simulink model "SS_Flyback_PLECS_Model_EVAL2"  (R2019b)
settings: Solver=VariableStepAuto  StartTime=0.0  StopTime=Ts  RelTol=1e-3
undefined symbols (not defined in the file or in its folder): fixed, plecs
libraries: plecslib_extras2 x1
settings Model: Creator=jbaxte24  LastModifiedBy=jb
settings DataIOCC: ReturnWorkspaceOutputs=off
settings DebuggingCC: ArithmeticOperatorsInVariantConditions=warning
settings SFSimCC: SimUseLocalCustomCode=off  CustomCodeUndefinedFunction=UseInterfaceOnly
settings RTWCC: RTWUseLocalCustomCode=off
settings CodeAppCC: StateflowObjectComments=on

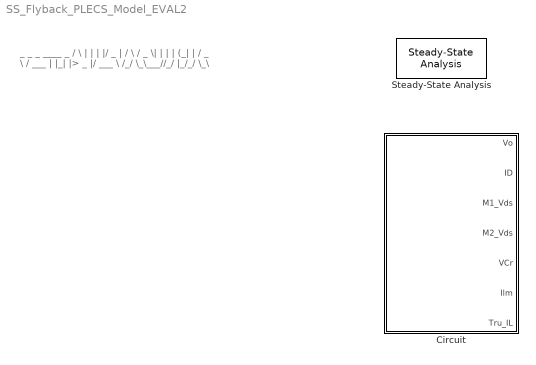
== system SS_Flyback_PLECS_Model_EVAL2 ==
  note: _ _ _ ____ _
      | / \ | | | |/ _ | / \
      | / _ \| | | | (_| | / _ \
      | / ___ | |_| |> _ |/ ___ \
      | /_/ \_\___//_/ |_/_/ \_\
  Circuit : Subsystem  LoadFcn=plecs('sl', 200);  InitFcn=plecs('sl', 214);  StartFcn=plecs('sl', 208);  StopFcn=plecs('sl', 209);  mask(PlecsCircuit){PLECSData=<binary blob, 3564 chars, not shown>}
      mask prompts: PLECSData "PLECS Data (Do not delete or modify!)"
      mask init:
      | % PLACE CUSTOM INITIALIZATIONS ABOVE
      | % DO NOT REMOVE
      | plecs('sl', 215);
      | % DO NOT REMOVE
      settings: CopyFcn=plecs('sl', 203);  DeleteFcn=plecs('sl', 205);  UndoDeleteFcn=plecs('sl', 206);  PreSaveFcn=plecs('sl', 211);  PostSaveFcn=plecs('sl', 201);  NameChangeFcn=plecs('sl', 210);  DestroyFcn=plecs('sl', 207);  PreCopyFcn=plecs('sl', 216);  OpenFcn=plecs('sl', 202);  ErrorFcn=plerrorfcn
      mask Help: web(['file:///' fullfile(plecsdoc, 'creatingacircuit.html')])
      mask Display: disp('PLECS\nCircuit')
  Steady-State Analysis : plecslib_extras2/Analysis Tools/Steady-State Analysis  Period=fixed  TriggerType=rising  TimeSpan=5e-06  TStart=0  MaxIter=10000  Tolerance=1e-6  Display=iteration  HideScopes=off  HiddenStates=error  FinalStateName=xSteadyState  NCycles=3  JPert=1e-4  JacobianCalculation=fast  NInitCycles=0
      settings: SourceProductName=PLECS Extras

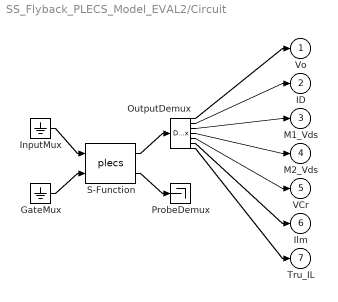
== system SS_Flyback_PLECS_Model_EVAL2/Circuit ==
  " GateMux " : Ground
  " InputMux " : Ground
  " OutputDemux " : Demux  Outputs=[ 1 1 1 1 1 1 1 ]
  " ProbeDemux " : Terminator
  " S-Function " : S-Function  FunctionName=plecs  SFunctionDeploymentMode=off  EnableBusSupport=off
  Vo : Outport  PortDimensions=1
  ID : Outport  Port=2  PortDimensions=1
  M1_Vds : Outport  Port=3  PortDimensions=1
  M2_Vds : Outport  Port=4  PortDimensions=1
  VCr : Outport  Port=5  PortDimensions=1
  Ilm : Outport  Port=6  PortDimensions=1
  Tru_IL : Outport  Port=7  PortDimensions=1
  wires:
  " InputMux "/1 -> " S-Function "/1
  " GateMux "/1 -> " S-Function "/2
  " S-Function "/1 -> " OutputDemux "/1
  " S-Function "/2 -> " ProbeDemux "/1
  " OutputDemux "/1 -> Vo/1
  " OutputDemux "/2 -> ID/1
  " OutputDemux "/3 -> M1_Vds/1
  " OutputDemux "/4 -> M2_Vds/1
  " OutputDemux "/5 -> VCr/1
  " OutputDemux "/6 -> Ilm/1
  " OutputDemux "/7 -> Tru_IL/1
